simulink model "Stabpendel"  (Simulink 7.1)
settings: Solver=ode45  StartTime=0.0  StopTime=4.0  RelTol=1e-3
settings Model: Creator=Meisel  LastModifiedBy=Meisel

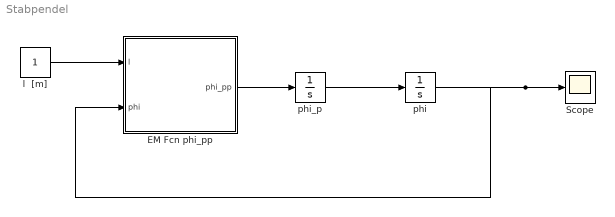
== system Stabpendel ==
  EM Fcn phi_pp : Stateflow chart
  Scope : Scope
  l  [m] : Constant  OutDataType=sfix(16)  OutScaling=2^0
  phi : Integrator  InitialCondition=30*pi/180
  phi_p : Integrator
  wires:
  phi_p/1 -> phi/1
  EM Fcn phi_pp/1(phi_pp) -> phi_p/1
  phi/1 -> EM Fcn phi_pp/2(phi), Scope/1
  l  [m]/1 -> EM Fcn phi_pp/1(l)

== matlab function EM Fcn phi_pp ==
  data: l input double; phi_pp output double; phi input double
function phi_pp = fcn(l, phi)
% Embedded MATLAB 

phi_pp = 3/2*9.81*sin(-phi)/l;
